simulink model "SegheriaSCADA"  (R2024b)
settings: Solver=FixedStepAuto  StartTime=0.0  StopTime=350  FixedStep=0.01  MaxStep=0.01  RelTol=1e-3
undefined symbols (not defined in the file or in its folder): b, b2, h, i_id, i_id2, i_max, kc, Kt, Kt2, Lt, Mag_D, Mag_legno, omega, omega2, SR, SR2, Tloss, Tloss2, w
libraries: simulink x3, slpidlib x2
settings Model: Creator=samue  LastModifiedBy=eliasantuari

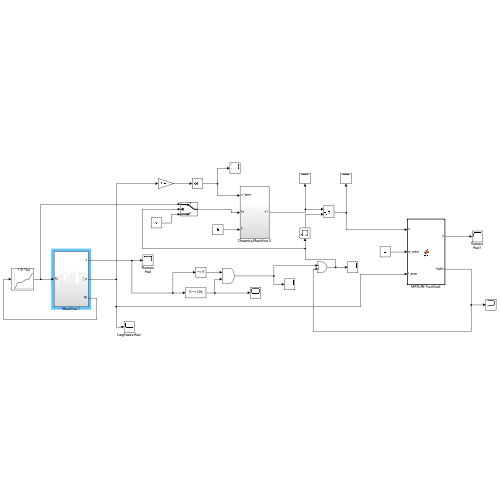
[thumbnail: Simulink's stored preview of the top-level diagram]
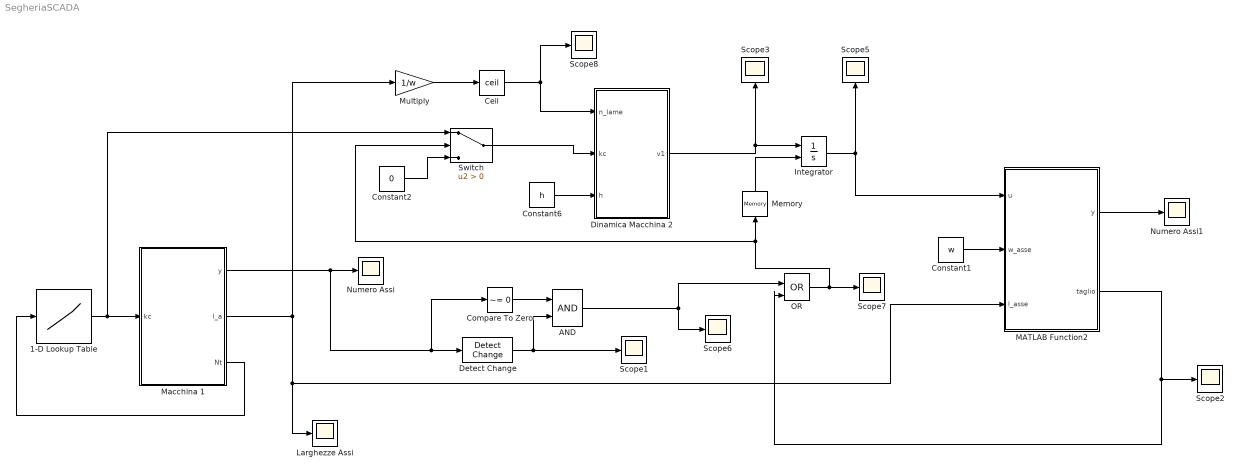
== system SegheriaSCADA ==
  1-D Lookup Table : Lookup_n-D  NumberOfTableDimensions=1  BreakpointsForDimension1=[0 1 2 3 4 5 ]  Table=kc  InternalRulePriority=Speed  RndMeth=Simplest
  AND : Logic  IconShape=distinctive  AllPortsSameDT=off  OutDataTypeStr=boolean
  Ceil : Rounding  Operator=ceil
  Compare To Zero : simulink/Logic and Bit Operations/Compare To Zero  relop=~=  OutDataTypeStr=boolean
  Constant1 : Constant  Value=w
  Constant2 : Constant  Value=0
  Constant6 : Constant  Value=h
  Detect Change : simulink/Logic and Bit Operations/Detect Change  vinit=0  OutDataTypeStr=boolean
  Dinamica Macchina 2 : Subsystem
  Integrator : Integrator  ExternalReset=falling
  Larghezze Assi : Scope
  MATLAB Function2 : MATLAB Function  TreatAsAtomicUnit=on
  Macchina 1 : Subsystem
  Memory : Memory
  Multiply : Gain  Gain=1/w
  Numero Assi : Scope
  Numero Assi1 : Scope
  OR : Logic  Operator=OR  IconShape=distinctive  AllPortsSameDT=off  OutDataTypeStr=boolean
  Scope{1..3,5..8} (7 alike) : Scope
  Switch : Switch  Criteria=u2 > Threshold  SaturateOnIntegerOverflow=off  InputSameDT=off
  wires:
  Macchina 1/1(y) -> Compare To Zero/1, Detect Change/1, Numero Assi/1
  Macchina 1/3(Nt) -> 1-D Lookup Table/1
  MATLAB Function2/1(y) -> Numero Assi1/1
  Constant1/1 -> MATLAB Function2/2(w_asse)
  Ceil/1 -> Dinamica Macchina 2/1(n_lame), Scope8/1
  Macchina 1/2(l_a) -> Larghezze Assi/1, MATLAB Function2/3(l_asse), Multiply/1
  Integrator/1 -> Scope5/1, MATLAB Function2/1(u)
  Constant6/1 -> Dinamica Macchina 2/3(h)
  1-D Lookup Table/1 -> Switch/1, Macchina 1/1(kc)
  Dinamica Macchina 2/1(v1) -> Scope3/1, Integrator/1
  Constant2/1 -> Switch/3
  Detect Change/1 -> Scope1/1, AND/2
  Switch/1 -> Dinamica Macchina 2/2(kc)
  Memory/1 -> Integrator/2
  MATLAB Function2/2(taglio) -> OR/2, Scope2/1
  Compare To Zero/1 -> AND/1
  AND/1 -> Scope6/1, OR/1
  Multiply/1 -> Ceil/1
  OR/1 -> Scope7/1, Switch/2, Memory/1

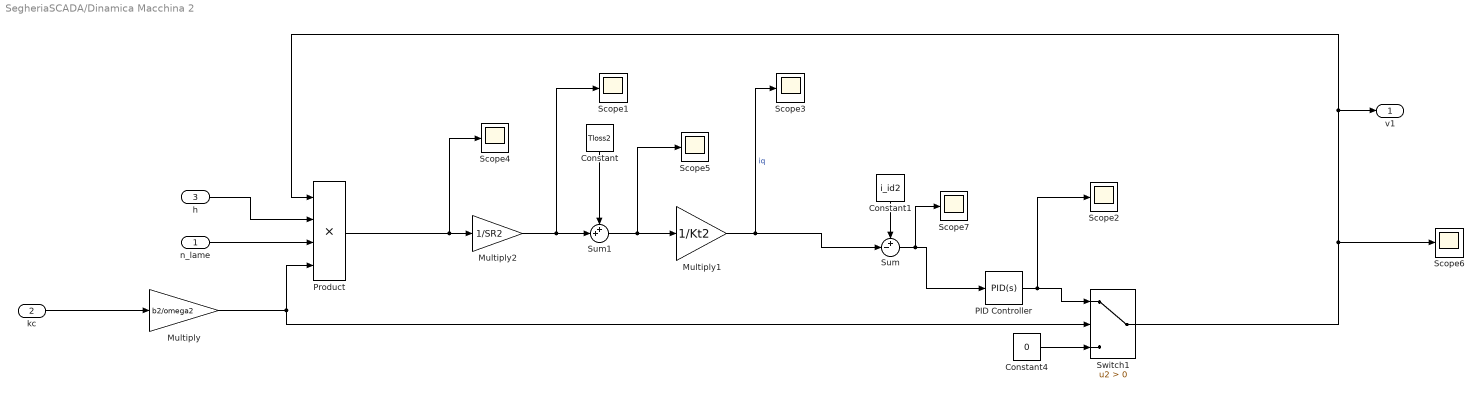
== system SegheriaSCADA/Dinamica Macchina 2 ==
  n_lame : Inport
  kc : Inport  Port=2
  h : Inport  Port=3
  Constant : Constant  Value=Tloss2
  Constant1 : Constant  Value=i_id2
  Constant4 : Constant  Value=0
  Multiply : Gain  Gain=b2/omega2
  Multiply1 : Gain  Gain=1/Kt2
  Multiply2 : Gain  Gain=1/SR2
  PID Controller : slpidlib/PID Controller  Controller=PID  Form=Parallel  TimeDomain=Continuous-time  UseExternalTs=off  SampleTime=-1  IntegratorMethod=Forward Euler  FilterMethod=Forward Euler  ControllerParametersSource=internal  P=0.3  I=0  UseKiTs=off  D=0  UseExternalDerivativeSource=off  N=100  UseFilter=on  TunerSelectOption=Transfer Function Based (PID Tuner App)  InitialConditionSource=internal  InitialConditionForIntegrator=0  InitialConditionForFilter=0  DifferentiatorICPrevScaledInput=0  ExternalReset=none  TrackingMode=off  Kt=1  LimitOutput=on  SatLimitsSource=internal  UpperSaturationLimit=60  LowerSaturationLimit=0  LinearizeAsGain=on  AntiWindupMode=none  Kb=1  LimitIntegrator=off  UpperIntegratorSaturationLimit=inf  LowerIntegratorSaturationLimit=-inf  POutMin=[]  POutMax=[]  IOutMin=[]  IOutMax=[]  DOutMin=[]  DOutMax=[]  NOutMin=[]  NOutMax=[]  SumOutMin=[]  SumOutMax=[]  SaturationOutMin=[]  SaturationOutMax=[]  PParamMin=[]  PParamMax=[]  IParamMin=[]  IParamMax=[]  DParamMin=[]  DParamMax=[]  NParamMin=[]  NParamMax=[]  KbParamMin=[]  KbParamMax=[]  KtParamMin=[]  KtParamMax=[]  KbOutMin=[]  KbOutMax=[]  KtOutMin=[]  KtOutMax=[]  IntegratorOutMin=[]  IntegratorOutMax=[]  FilterOutMin=[]  FilterOutMax=[]  SumI1OutMin=[]  SumI1OutMax=[]  SumI2OutMin=[]  SumI2OutMax=[]  SumI3OutMin=[]  SumI3OutMax=[]  SumI4OutMin=[]  SumI4OutMax=[]  SumDOutMin=[]  SumDOutMax=[]  DifferentiatorOutMin=[]  DifferentiatorOutMax=[]  FilterDiffOutCoefMin=[]  FilterDiffOutCoefMax=[]  ReciprocalOutMin=[]  ReciprocalOutMax=[]  SumDenOutMin=[]  SumDenOutMax=[]  SumNumOutMin=[]  SumNumOutMax=[]  DivideOutMin=[]  DivideOutMax=[]  UdiffTsProdOutMin=[]  UdiffTsProdOutMax=[]  NTsProdOutMin=[]  NTsProdOutMax=[]  UintegralTsProdOutMin=[]  UintegralTsProdOutMax=[]  UngainTsProdOutMin=[]  UngainTsProdOutMax=[]  ClampingZeroOutDataTypeStr=Inherit: Inherit via back propagation  ClampingZeroOutMin=[]  ClampingZeroOutMax=[]  FilterDenConstantOutDataTypeStr=Inherit: Inherit via back propagation  FilterDenConstantOutMin=[]  FilterDenConstantOutMax=[]  PCopyOutDataTypeStr=Inherit: Inherit via back propagation  PCopyOutMin=[]  PCopyOutMax=[]  NCopyOutDataTypeStr=Inherit: Inherit via back propagation  NCopyOutMin=[]  NCopyOutMax=[]  IntegratorContinuousStateAttributes=''  IntegratorStateMustResolveToSignalObject=off  IntegratorRTWStateStorageClass=Auto  FilterContinuousStateAttributes=''  FilterStateMustResolveToSignalObject=off  FilterRTWStateStorageClass=Auto  ParallelPVariant=InternalParameters  IdealPVariant=Disabled  IVariant=InternalParameters  DVariant=InternalParameters  IntegratorVariant=Continuous  SatVariant=Enabled  AWVariant=Passthrough  PCopyVariant=Disabled  TRVariant=Disabled  FdbkBlocksVariant=Forward  IdealPFdbkVariant=Disabled  SatFdbkVariant=Disabled  DerivativeFilterVariant=ContFilter  NVariant=InternalParameters  NCopyVariant=Disabled  FilterICVariant=InternalICsFilter  IntegratorICVariant=InternalICs  ExternalResetVariant=Disabled  TRSumVariant=Passthrough  SumFdbkVariant=Disabled  SumVariant=Sum_PID  TsampFilterVariant=InternalTs  TsampNgainVariant=Passthrough  TsampIntegralVariant=Disabled_SignalSpec  ExternalSaturationOutDataTypeStr=Inherit: Same as second input  DerivativeSourceVariant=ErrorSignal  PreIntVariant=InternalPreInt
  Product : Product  Inputs=4
  Scope{1..7} (7 alike) : Scope
  Sum : Sum  Inputs=+-|
  Sum1 : Sum  Inputs=++|
  Switch1 : Switch  Criteria=u2 > Threshold  SaturateOnIntegerOverflow=off  InputSameDT=off
  v1 : Outport
  wires:
  Constant4/1 -> Switch1/3
  Product/1 -> Scope4/1, Multiply2/1
  PID Controller/1 -> Scope2/1, Switch1/1
  Multiply1/1 -> Sum/2, Scope3/1  "iq"
  Multiply/1 -> Switch1/2, Product/4
  kc/1 -> Multiply/1
  Constant1/1 -> Sum/1
  Sum/1 -> Scope7/1, PID Controller/1
  Multiply2/1 -> Scope1/1, Sum1/2
  Sum1/1 -> Scope5/1, Multiply1/1
  Constant/1 -> Sum1/1
  h/1 -> Product/2
  n_lame/1 -> Product/3
  Switch1/1 -> Scope6/1, Product/1, v1/1

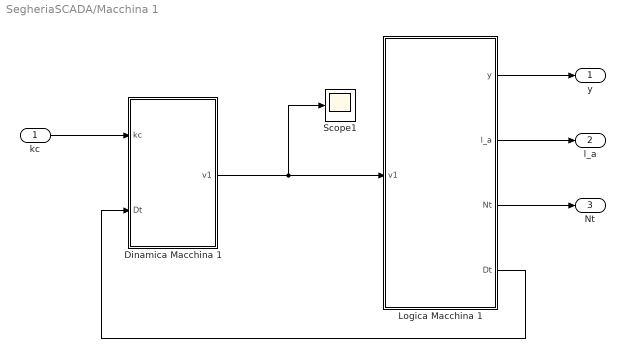
== system SegheriaSCADA/Macchina 1 ==
  kc : Inport
  Dinamica Macchina 1 : Subsystem
  Logica Macchina 1 : Subsystem
  Scope1 : Scope
  y : Outport
  l_a : Outport  Port=2
  Nt : Outport  Port=3
  wires:
  kc/1 -> Dinamica Macchina 1/1(kc)
  Dinamica Macchina 1/1(v1) -> Scope1/1, Logica Macchina 1/1(v1)
  Logica Macchina 1/3(Nt) -> Nt/1
  Logica Macchina 1/4(Dt) -> Dinamica Macchina 1/2(Dt)
  Logica Macchina 1/1(y) -> y/1
  Logica Macchina 1/2(l_a) -> l_a/1

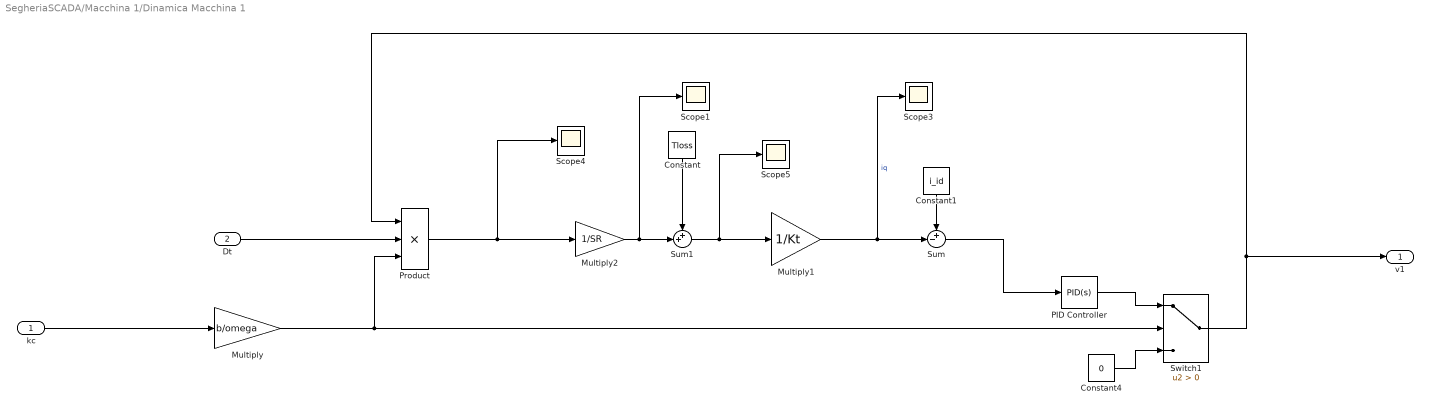
== system SegheriaSCADA/Macchina 1/Dinamica Macchina 1 ==
  kc : Inport
  Dt : Inport  Port=2
  Constant : Constant  Value=Tloss
  Constant1 : Constant  Value=i_id
  Constant4 : Constant  Value=0
  Multiply : Gain  Gain=b/omega
  Multiply1 : Gain  Gain=1/Kt
  Multiply2 : Gain  Gain=1/SR
  PID Controller : slpidlib/PID Controller  Controller=PID  Form=Parallel  TimeDomain=Continuous-time  UseExternalTs=off  SampleTime=-1  IntegratorMethod=Forward Euler  FilterMethod=Forward Euler  ControllerParametersSource=internal  P=0  I=0.0048685791703887  UseKiTs=off  D=0  UseExternalDerivativeSource=off  N=100  UseFilter=on  TunerSelectOption=Transfer Function Based (PID Tuner App)  InitialConditionSource=internal  InitialConditionForIntegrator=0  InitialConditionForFilter=0  DifferentiatorICPrevScaledInput=0  ExternalReset=none  TrackingMode=off  Kt=1  LimitOutput=off  SatLimitsSource=internal  UpperSaturationLimit=i_max  LowerSaturationLimit=-inf  LinearizeAsGain=on  AntiWindupMode=none  Kb=1  LimitIntegrator=off  UpperIntegratorSaturationLimit=inf  LowerIntegratorSaturationLimit=-inf  POutMin=[]  POutMax=[]  IOutMin=[]  IOutMax=[]  DOutMin=[]  DOutMax=[]  NOutMin=[]  NOutMax=[]  SumOutMin=[]  SumOutMax=[]  SaturationOutMin=[]  SaturationOutMax=[]  PParamMin=[]  PParamMax=[]  IParamMin=[]  IParamMax=[]  DParamMin=[]  DParamMax=[]  NParamMin=[]  NParamMax=[]  KbParamMin=[]  KbParamMax=[]  KtParamMin=[]  KtParamMax=[]  KbOutMin=[]  KbOutMax=[]  KtOutMin=[]  KtOutMax=[]  IntegratorOutMin=[]  IntegratorOutMax=[]  FilterOutMin=[]  FilterOutMax=[]  SumI1OutMin=[]  SumI1OutMax=[]  SumI2OutMin=[]  SumI2OutMax=[]  SumI3OutMin=[]  SumI3OutMax=[]  SumI4OutMin=[]  SumI4OutMax=[]  SumDOutMin=[]  SumDOutMax=[]  DifferentiatorOutMin=[]  DifferentiatorOutMax=[]  FilterDiffOutCoefMin=[]  FilterDiffOutCoefMax=[]  ReciprocalOutMin=[]  ReciprocalOutMax=[]  SumDenOutMin=[]  SumDenOutMax=[]  SumNumOutMin=[]  SumNumOutMax=[]  DivideOutMin=[]  DivideOutMax=[]  UdiffTsProdOutMin=[]  UdiffTsProdOutMax=[]  NTsProdOutMin=[]  NTsProdOutMax=[]  UintegralTsProdOutMin=[]  UintegralTsProdOutMax=[]  UngainTsProdOutMin=[]  UngainTsProdOutMax=[]  ClampingZeroOutDataTypeStr=Inherit: Inherit via back propagation  ClampingZeroOutMin=[]  ClampingZeroOutMax=[]  FilterDenConstantOutDataTypeStr=Inherit: Inherit via back propagation  FilterDenConstantOutMin=[]  FilterDenConstantOutMax=[]  PCopyOutDataTypeStr=Inherit: Inherit via back propagation  PCopyOutMin=[]  PCopyOutMax=[]  NCopyOutDataTypeStr=Inherit: Inherit via back propagation  NCopyOutMin=[]  NCopyOutMax=[]  IntegratorContinuousStateAttributes=''  IntegratorStateMustResolveToSignalObject=off  IntegratorRTWStateStorageClass=Auto  FilterContinuousStateAttributes=''  FilterStateMustResolveToSignalObject=off  FilterRTWStateStorageClass=Auto  ParallelPVariant=InternalParameters  IdealPVariant=Disabled  IVariant=InternalParameters  DVariant=InternalParameters  IntegratorVariant=Continuous  SatVariant=Disabled  AWVariant=Passthrough  PCopyVariant=Disabled  TRVariant=Disabled  FdbkBlocksVariant=Forward  IdealPFdbkVariant=Disabled  SatFdbkVariant=Disabled  DerivativeFilterVariant=ContFilter  NVariant=InternalParameters  NCopyVariant=Disabled  FilterICVariant=InternalICsFilter  IntegratorICVariant=InternalICs  ExternalResetVariant=Disabled  TRSumVariant=Passthrough  SumFdbkVariant=Disabled  SumVariant=Sum_PID  TsampFilterVariant=InternalTs  TsampNgainVariant=Passthrough  TsampIntegralVariant=Disabled_SignalSpec  ExternalSaturationOutDataTypeStr=Inherit: Same as second input  DerivativeSourceVariant=ErrorSignal  PreIntVariant=InternalPreInt
  Product : Product  Inputs=3
  Scope{1,3..5} (4 alike) : Scope
  Sum : Sum  Inputs=+-|
  Sum1 : Sum  Inputs=++|
  Switch1 : Switch  Criteria=u2 > Threshold  SaturateOnIntegerOverflow=off  InputSameDT=off
  v1 : Outport
  wires:
  Constant4/1 -> Switch1/3
  Product/1 -> Scope4/1, Multiply2/1
  PID Controller/1 -> Switch1/1
  Multiply1/1 -> Scope3/1, Sum/2  "iq"
  Multiply/1 -> Product/3, Switch1/2
  kc/1 -> Multiply/1
  Switch1/1 -> v1/1, Product/1
  Constant1/1 -> Sum/1
  Sum/1 -> PID Controller/1
  Multiply2/1 -> Scope1/1, Sum1/2
  Sum1/1 -> Scope5/1, Multiply1/1
  Constant/1 -> Sum1/1
  Dt/1 -> Product/2

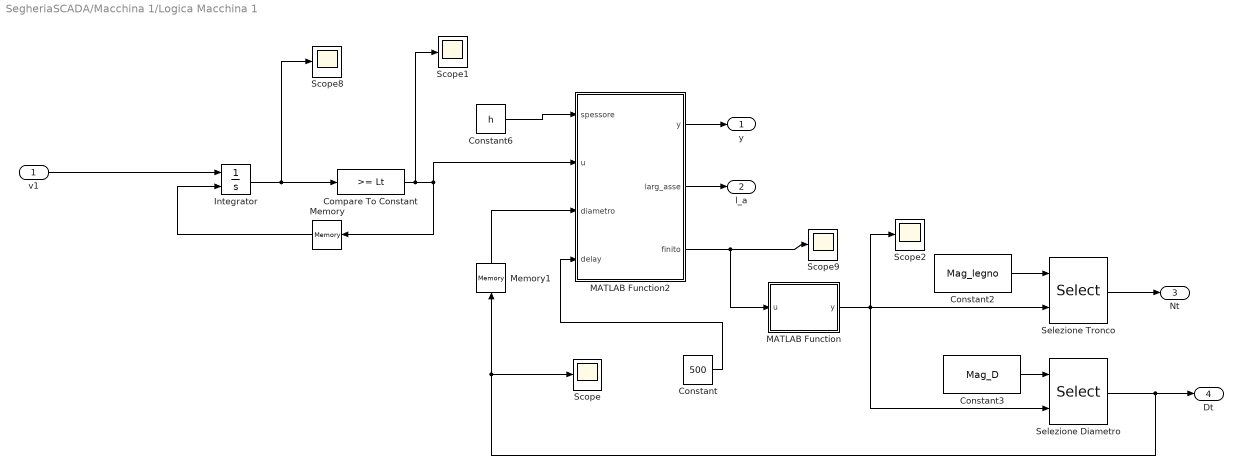
== system SegheriaSCADA/Macchina 1/Logica Macchina 1 ==
  v1 : Inport
  Compare To Constant : simulink/Logic and Bit Operations/Compare To Constant  relop=>=  const=Lt  OutDataTypeStr=boolean
  Constant : Constant  Value=500
  Constant2 : Constant  Value=Mag_legno
  Constant3 : Constant  Value=Mag_D
  Constant6 : Constant  Value=h
  Integrator : Integrator  ExternalReset=rising
  MATLAB Function : MATLAB Function  TreatAsAtomicUnit=on
  MATLAB Function2 : MATLAB Function  TreatAsAtomicUnit=on
  Memory : Memory
  Memory1 : Memory
  Scope{,1..2,8..9} (5 alike) : Scope
  Selezione Diametro : Selector  IndexMode=Zero-based  InputPortWidth=length(Mag_D)  IndexOptions=Index vector (port)  Indices=[1 3]  OutputSizes=1
  Selezione Tronco : Selector  IndexMode=Zero-based  InputPortWidth=length(Mag_legno)  IndexOptions=Index vector (port)  Indices=[1 3]  OutputSizes=1
  y : Outport
  l_a : Outport  Port=2
  Nt : Outport  Port=3
  Dt : Outport  Port=4
  wires:
  Constant6/1 -> MATLAB Function2/1(spessore)
  MATLAB Function2/3(finito) -> Scope9/1, MATLAB Function/1(u)
  Memory/1 -> Integrator/2
  Memory1/1 -> MATLAB Function2/3(diametro)
  Constant2/1 -> Selezione Tronco/1
  v1/1 -> Integrator/1
  Integrator/1 -> Compare To Constant/1, Scope8/1
  Constant3/1 -> Selezione Diametro/1
  MATLAB Function/1(y) -> Selezione Diametro/2, Scope2/1, Selezione Tronco/2
  MATLAB Function2/1(y) -> y/1
  Selezione Tronco/1 -> Nt/1
  MATLAB Function2/2(larg_asse) -> l_a/1
  Compare To Constant/1 -> Scope1/1, Memory/1, MATLAB Function2/2(u)
  Selezione Diametro/1 -> Dt/1, Memory1/1, Scope/1
  Constant/1 -> MATLAB Function2/4(delay)

== matlab function SegheriaSCADA/MATLAB Function2 ==
  settings: updateMethod=DISCRETE
  data: u input; w_asse input; y output; l_asse input; taglio output; Lt parameter
function [y, taglio] = fcn(u, w_asse, l_asse, Lt)
    persistent counter 

    n_assi = floor(l_asse / w_asse);
    
    taglio = 0;

    if isempty(counter)
        counter = 0;
    end

    % Conto assi tagliate
    if u >= Lt
        counter = counter + n_assi;
    end

    % Segnale di taglio
    if  (u > 0 && u < Lt && l_asse > 0) 
        taglio = 1;
    end

    y = counter;
end

== matlab function SegheriaSCADA/Macchina 1/Logica Macchina 1/MATLAB Function ==
  data: u input; y output; Mag_legno parameter
function y = fcn(u, Mag_legno)
    persistent counter
    if isempty(counter)
        counter = 0;
    end

    if u == 1
        counter = counter + 1;
    end

    y = counter;
    
    if y > length(Mag_legno)-1
        y = 0;
    end

end

== matlab function SegheriaSCADA/Macchina 1/Logica Macchina 1/MATLAB Function2 ==
  settings: updateMethod=DISCRETE
  data: spessore input; u input; y output; diametro input; larg_asse output; finito output; delay input
function [y, larg_asse, finito] = fcn(spessore, u, diametro, delay)

persistent counter delay_count state 

% state:
% 0 = conteggio tagli
% 1 = attesa tra 5 e 6
% 2 = impulso 6
% 3 = reset

if isempty(counter)
    counter = 0;
    delay_count = 0;
    state = 0;
end

max_assi  = floor(diametro / spessore);  % es. 6
max_tagli = max_assi - 1;                % es. 5

finito = 0;

switch state
    
    % =============================
    case 0   % Conteggio tagli reali
    % =============================
        if u == 1
            counter = counter + 1;
        end
        
        if counter >= max_tagli
            counter = max_tagli;  % resta a 5
            state = 1;
            delay_count = 0;
        end
        
    % =============================
    case 1   % Attesa tra 5 e 6
    % =============================
        delay_count = delay_count + 1;
        
        if delay_count >= delay
            state = 2;
        end
        
    % =============================
    case 2   % Impulso asse finale
    % =============================
        counter = max_assi;   % 6
        finito = 1;
        state = 3;

        
    % =============================
    case 3   % Reset
    % =============================
        counter = 0;
        state = 0;
        
end

% =============================
% Calcolo larghezza asse
% =============================


distanza_bordo = counter * spessore;
   
h = abs(diametro/2 - distanza_bordo + spessore/2);

arg = (diametro/2)^2 - h^2;
arg = max(arg, 0);   % evita errori sqrt
    
larg_asse = 2 * sqrt(arg);


y = counter;
